simulink model "legoSS_MCC_sim (1)"  (R2025a)
settings: Solver=ode45  StartTime=0.0  StopTime=10.0  RelTol=1e-3  EnableMultiTasking=on
values from neighbouring files (symbols this model uses):
  A = compan(cell2mat(TF_U_theta.Denominator))    [Asservissement_moteur.m]    (also in Test.m = [0 1;-denom(3) -denom(2)])
  B = [1 0]'    [Asservissement_moteur.m]    (also in Test.m = [num(2) num(3)]')
settings Model: Creator=jacques  LastModifiedBy=carol
settings SolverCC: AlgebraicLoopSolver=TrustRegion
settings DataIOCC: LimitDataPoints=on  SaveFormat=Array  SignalLoggingSaveFormat=ModelDataLogs  ReturnWorkspaceOutputs=off
settings OptimizationCC: ExpressionDepthLimit=2147483647.0  LifeSpan=inf
settings DebuggingCC: UnderspecifiedInitializationDetection=Classic  MergeDetectMultiDrivingBlocksExec=none  SolverPrmCheckMsg=warning  FcnCallInpInsideContextMsg=warning  UnconnectedInputMsg=warning  UnconnectedOutputMsg=warning  UnconnectedLineMsg=warning  StateNameClashWarn=warning  SFUnexpectedBacktrackingDiag=warning  SFNoUnconditionalDefaultTransitionDiag=warning  SFExecutionAtInitializationDiag=none  ArithmeticOperatorsInVariantConditions=warning
settings HardwareCC: ProdBitPerPointer=32.0  ProdBitPerSizeT=32.0  ProdBitPerPtrDiffT=32.0  ProdLargestAtomicFloat=None  ProdIntDivRoundTo=Undefined  ProdEndianess=Unspecified  ProdWordSize=32.0  ProdHWDeviceType=32-bit Generic
settings ModelReferenceCC: EnableRefExpFcnMdlSchedulingChecks=on  PropagateSignalLabelsOutOfModel=off
settings SFSimCC: SimUseLocalCustomCode=off  CustomCodeUndefinedFunction=UseInterfaceOnly
settings RTWCC: RTWUseLocalCustomCode=off  GPUComputeCapability=3.5  DLArmComputeVersion=19.05
settings CodeAppCC: StateflowObjectComments=on
settings GRTTargetCC: TargetLangStandard=C89/C90 (ANSI)  CombineOutputUpdateFcns=off  GRTInterface=on
settings ConfigComp: CovMetricSettings=dw  CovSaveCumulativeToWorkspaceVar=on  CovSaveSingleToWorkspaceVar=on  CovExternalEMLEnable=off

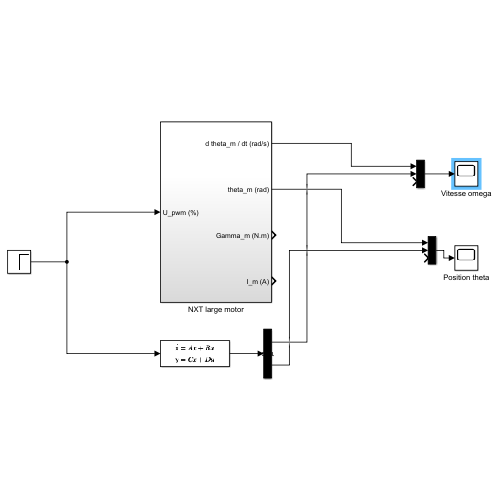
[thumbnail: Simulink's stored preview of the top-level diagram]
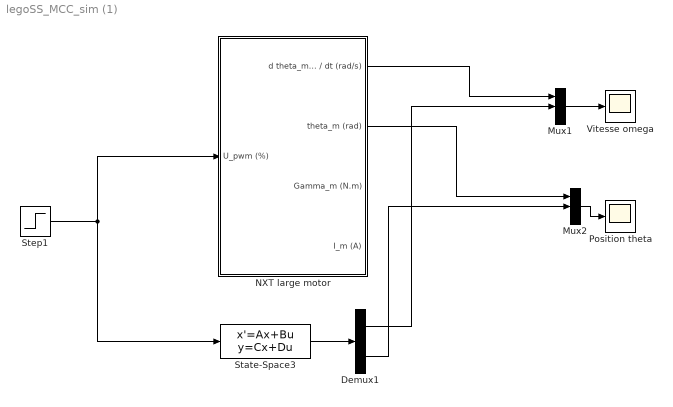
== system legoSS_MCC_sim (1) ==
  Demux1 : Demux  Outputs=2
      settings: DisplayOption=none
  Mux1 : Mux  Inputs=3
  Mux2 : Mux  Inputs=3
  NXT large motor : Subsystem
  Position theta : Scope
      settings: ActiveDisplayYMinimum=-0.15627655520727263  ActiveDisplayYMaximum=1.4064889968654539
  State-Space3 : StateSpace  A=A  B=B  C=[0,1;1,0]  D=zeros(2,1)  InitialCondition=0
  Step1 : Step  SampleTime=0
  Vitesse omega : Scope
      settings: ActiveDisplayYMinimum=-0.017455700065657442  ActiveDisplayYMaximum=0.157101300590917
  wires:
  Step1/1 -> NXT large motor/1(U_pwm (%)), State-Space3/1
  State-Space3/1 -> Demux1/1
  NXT large motor/1(d theta_m / dt (rad/s)) -> Mux1/1
  Mux1/1 -> Vitesse omega/1
  NXT large motor/2(theta_m (rad)) -> Mux2/1
  Mux2/1 -> Position theta/1
  Demux1/1 -> Mux1/2
  Demux1/2 -> Mux2/2

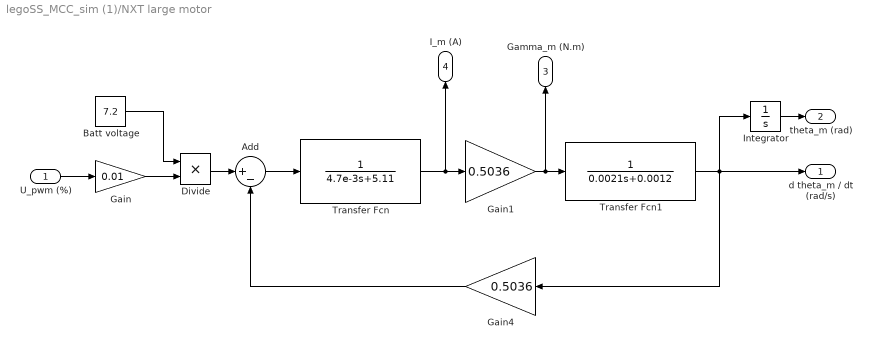
== system legoSS_MCC_sim (1)/NXT large motor ==
  U_pwm (%) : Inport
  Add : Sum  Inputs=|+-
  Batt voltage : Constant  Value=7.2
  Divide : Product  Inputs=**
  Gain : Gain  Gain=0.01
  Gain1 : Gain  Gain=0.5036
  Gain4 : Gain  Gain=0.5036
  Integrator : Integrator
  Transfer Fcn : TransferFcn  Denominator=[4.7e-3 5.11]
  Transfer Fcn1 : TransferFcn  Denominator=[0.0021 0.0012]
  d theta_m / dt (rad/s) : Outport
  theta_m (rad) : Outport  Port=2
  Gamma_m (N.m) : Outport  Port=3
  I_m (A) : Outport  Port=4
  wires:
  Batt voltage/1 -> Divide/1
  Gain/1 -> Divide/2
  Divide/1 -> Add/1
  Add/1 -> Transfer Fcn/1
  Transfer Fcn/1 -> Gain1/1, I_m (A)/1
  Gain1/1 -> Transfer Fcn1/1, Gamma_m (N.m)/1
  Transfer Fcn1/1 -> Integrator/1, Gain4/1, d theta_m / dt (rad/s)/1
  Gain4/1 -> Add/2
  U_pwm (%)/1 -> Gain/1
  Integrator/1 -> theta_m (rad)/1
